simulink model "simModel"  (R2018a)
settings: Solver=FixedStepDiscrete  StartTime=0.0  StopTime=10.0  FixedStep=0.05  RelTol=1e-3
undefined symbols (not defined in the file or in its folder): gray
settings Model: Creator=aoki-soya  LastModifiedBy=aoki-soya

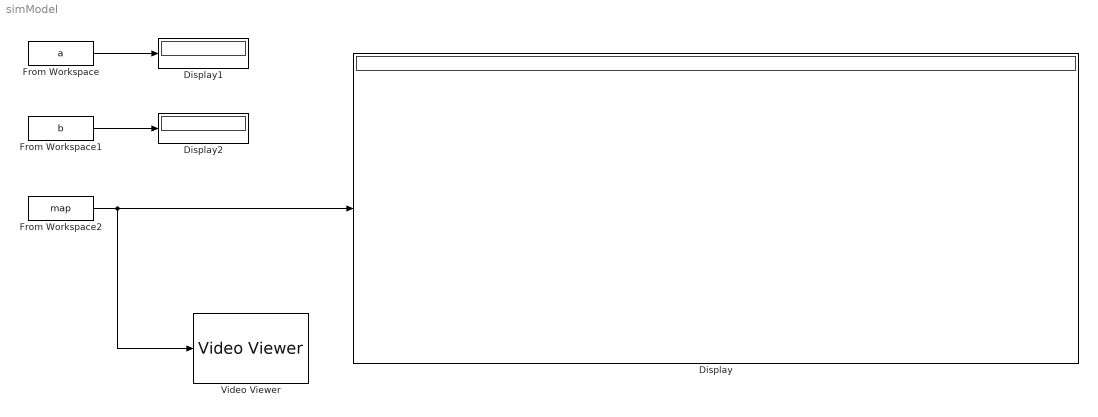
== system simModel ==
  Display : Display
  Display1 : Display
  Display2 : Display
  From Workspace : FromWorkspace  VariableName=a  SampleTime=0  OutputAfterFinalValue=Holding final value
  From Workspace1 : FromWorkspace  VariableName=b  SampleTime=0  OutputAfterFinalValue=Holding final value
  From Workspace2 : FromWorkspace  VariableName=map  SampleTime=0  OutputAfterFinalValue=Holding final value
  Video Viewer : VideoViewer  colormapValue=gray(256)  FigPos=[1 1198 859 247]
  wires:
  From Workspace2/1 -> Video Viewer/1, Display/1
  From Workspace/1 -> Display1/1
  From Workspace1/1 -> Display2/1
